simulink model "Ueberholmanoever_david"  (R2018a)
settings: Solver=ode1  StartTime=0.0  StopTime=inf  FixedStep=1/10  RelTol=1e-3  EnableMultiTasking=on
undefined symbols (not defined in the file): finding, gray, Lane, PiCar_library, Rec, SDTV
libraries: simulink x15, visiontextngfix x2, visiontransforms x2, visionconversions x1, visionanalysis x1, visionstatistics x1, embdlinuxlib x1
(part 2 of 2)

== matlab function Ueberholmanoever_david/Lane-finding/MATLAB Function ==
  data: planecoords output; theta output; points input; dist_real output
function [planecoords, theta, dist_real]  = CamToWorld(points)

pixelcoords = zeros(2,2);
pixelcoords(1,:) = points(1,1:2);
pixelcoords(2,:) = points(1,3:4);


pos = zeros(2,3);
alpha = 19.5 * pi / 180;

for i = 1:1:2
    pixelcoord = pixelcoords(i,:);
    pixelcoord(1) = pixelcoord(1) * 4;
    pixelcoord(2) =  pixelcoord(2) + 150;
    plane_height = 0;  %77 bei Iske Buch
    %alpha = 18.5; %18.5
    h= 275 - plane_height;
    f_px =[276.3065;275.7723];
    image_size = [320;240];
    camera_pos = [0;275;-315];

    %Pixelkoordinatensystem verschieben
    pixelcoord(1) = pixelcoord(1) - image_size(1)/2;
    pixelcoord(2) = -pixelcoord(2) + image_size(2)/2;

    %pixelcoords(i,:) = pixelcoord;
    
    %Position sch?tzen
    
    z_est = h/cos(alpha) / (tan(alpha) - pixelcoord(2)/f_px(2));
    y_est = z_est * pixelcoord(2)/f_px(2);
    x_est = z_est * pixelcoord(1)/f_px(1);

    %rotieren
    pos1 = [1 0 0; 0 cos(alpha) -sin(alpha); 0 sin(alpha) cos(alpha)] * [x_est; y_est; z_est];

    %Position der Kamera einbeziehen
    pos(i,:) = pos1 + camera_pos; 
    
end

planecoords = zeros(2,2);
planecoords = pos(:,1:2:3);

x_diff = planecoords(1,1) - planecoords(2,1);
y_diff = planecoords(1,2) - planecoords(2,2);

theta = 0;
theta = atan(x_diff / y_diff);
theta = theta *180 / pi;

dist_real = 0;
v1 = [planecoords(1,1),0,planecoords(1,2)];
v2 = [planecoords(2,1),0,planecoords(2,2)];
a = v1 - v2;
b = -v2;
dist_real = sign(planecoords(2,1)) * sqrt(sum(cross(a,b,2).^2,2)) ./sqrt(sum(a.^2,2));

== matlab function Ueberholmanoever_david/Switch Case Action Subsystem4/CamToWorld ==
  data: pixelcoord input; pos output
%CamToWorld([0;0], 10/180*pi, 150, 5);
%alpha in grad
function pos  = CamToWorld(pixelcoord)
plane_height = 72; %179 oben am vorderen auto    %72; %box auf boden  %77 bei Iske Buch
alpha = 18.5; %18.5
h= 275 - plane_height;
f_px =[276.3065;275.7723];
image_size = [320;240];
camera_pos = [0;275;-315];

%Pixelkoordinatensystem verschieben
pixelcoord(1) = pixelcoord(1) - image_size(1)/2;
pixelcoord(2) = -pixelcoord(2) + image_size(2)/2;

%Position sch?tzen
alpha = alpha * pi / 180;
z_est = h/cos(alpha) / (tan(alpha) - pixelcoord(2)/f_px(2));
y_est = z_est * pixelcoord(2)/f_px(2);
x_est = z_est * pixelcoord(1)/f_px(1);

%rotieren
pos1 = [1 0 0; 0 cos(alpha) -sin(alpha); 0 sin(alpha) cos(alpha)] * [x_est; y_est; z_est];

%Position der Kamera einbeziehen
pos = pos1 + camera_pos;


end

== matlab function Ueberholmanoever_david/Switch Case Action Subsystem4/RedRectangleDetection ==
  data: I input; pts output; max output
function [pts,max]  = objectDet(I)


red = I(:,:,1);
green = I(:,:,2);
blue = I(:,:,3);

red2 = double(red);
green2 = double(green);
blue2 = double(blue);
%out = red > 200 & red < 250 & green > 40 & green < 150 & blue > 90 & blue < 200;

%out = red > 115 & red < 160 & green > 25 & green < 55 & blue > 15 & blue < 40;
out = (100*red2) > (50 * (red2 + green2 + blue2)) & (red2 + green2 + blue2) > 120;



centr = regionprops(out,'centroid');
area = regionprops(out,'area');

area2 = struct2cell(area);
max = 0;
idx = 0;
for i = 1:1:length(area2)
if area2{1,i} > max 
max = area2{1,i};
idx = i;
end
end
if max == 0
y1 = length(red(:,1))/2;
x1 = length(red(1,:))/2;
else
help = struct2cell(centr(idx));
x1 = help{1,1}(1);
y1 = help{1,1}(2);
end
pts = [x1,y1,1];
end

== matlab function Ueberholmanoever_david/Switch Case Action Subsystem4/calcDistance  ==
  data: desired_pos input; world_coords input; dist_x output; dist_z output
function [dist_x,dist_z] = calcDistance(desired_pos,world_coords)

dist_x = world_coords(1) - desired_pos(1)-30;  % dist from the centre of the image, for steering
dist_z = world_coords(3) - desired_pos(2);  % dist from the car

% if (dist_z > 0)
%     speed = 100;
% else
%     speed = -600;
% end   
end
